simulink model "EnabledSubSystem4Blocks"  (Simulink 7.6)
settings: Solver=ode45  StartTime=0.0  StopTime=10.0  RelTol=1e-3
settings Model: Creator=DominikC  LastModifiedBy=DominikC
settings DebuggingCC: FcnCallInpInsideContextMsg=Enable All

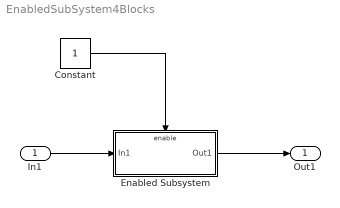
== system EnabledSubSystem4Blocks ==
  In1 : Inport
  Constant : Constant
  Enabled Subsystem : Subsystem  TreatAsAtomicUnit=on
  Out1 : Outport
  wires:
  In1/1 -> Enabled Subsystem/1(In1)
  Enabled Subsystem/1(Out1) -> Out1/1
  Constant/1 -> Enabled Subsystem/Enable

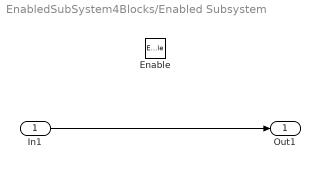
== system EnabledSubSystem4Blocks/Enabled Subsystem ==
  In1 : Inport
  Enable : EnablePort
  Out1 : Outport
  wires:
  In1/1 -> Out1/1
